simulink model "fft_block_3_19"  (R2023a)
settings: Solver=VariableStepAuto  StartTime=0.0  StopTime=1024*20  RelTol=1e-3
libraries: hdlsllib x7, dsphdlxfrm2 x2, HDLMathLib x2, simulink x1
settings Model: Creator=75549  LastModifiedBy=19595
settings ModelReferenceCC: EnableRefExpFcnMdlSchedulingChecks=on

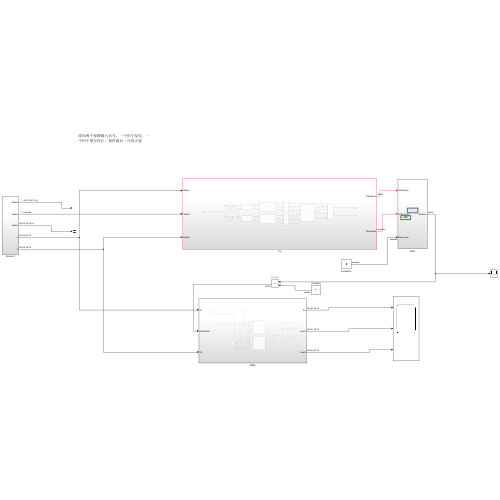
[thumbnail: Simulink's stored preview of the top-level diagram]
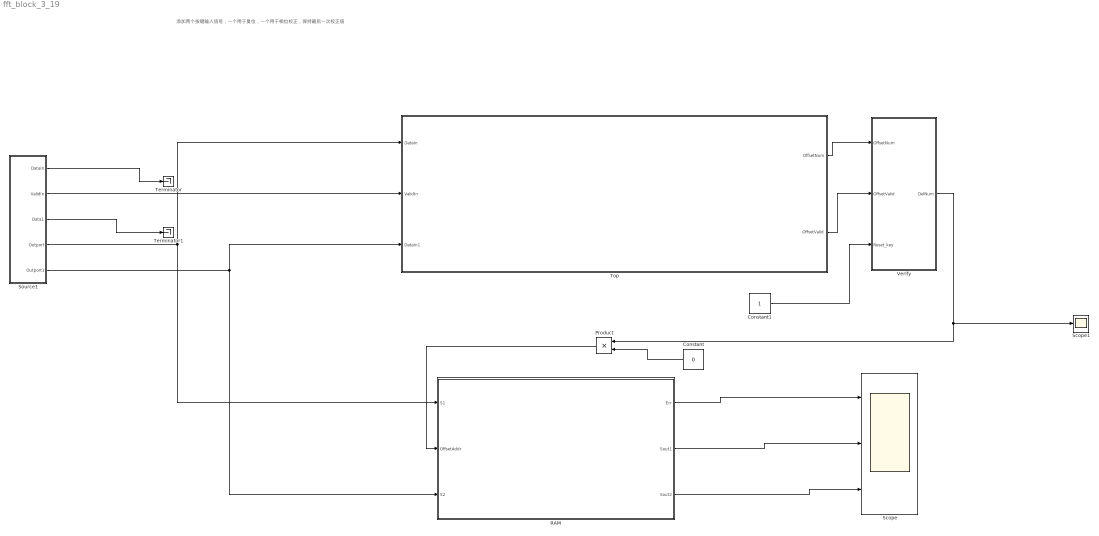
== system fft_block_3_19 ==
  note: 添加两个按键输入信号，一个用于复位，一个用于相位校正，保持最后一次校正值
  Constant : Constant  Value=0  VectorParams1D=off  SampleTime=-1
  Constant1 : Constant  VectorParams1D=off  OutDataTypeStr=boolean  SampleTime=-1
  Product : Product  OutDataTypeStr=uint16
  RAM : Subsystem
  Scope : Scope  NumInputPorts=3
  Scope1 : Scope
  Source1 : Subsystem
  Terminator : Terminator
  Terminator1 : Terminator
  Top : Subsystem
  Verify : Subsystem
  wires:
  Verify/1(DelNum) -> Product/1, Scope1/1
  RAM/2(Sout1) -> Scope/2
  Source1/4(Outport) -> Top/1(DataIn), RAM/1(S1)
  Source1/2(ValidIn) -> Top/2(ValidIn)
  Top/2(OffsetValid) -> Verify/2(OffsetValid)
  Top/1(OffsetNum) -> Verify/1(OffsetNum)
  Source1/1(DataIn) -> Terminator/1
  Source1/3(Data1) -> Terminator1/1
  RAM/1(Err) -> Scope/1
  Source1/5(Outport1) -> Top/3(DataIn1), RAM/3(S2)
  RAM/3(Sout2) -> Scope/3
  Constant/1 -> Product/2
  Product/1 -> RAM/2(OffsetAddr)
  Constant1/1 -> Verify/3(Reset_key)

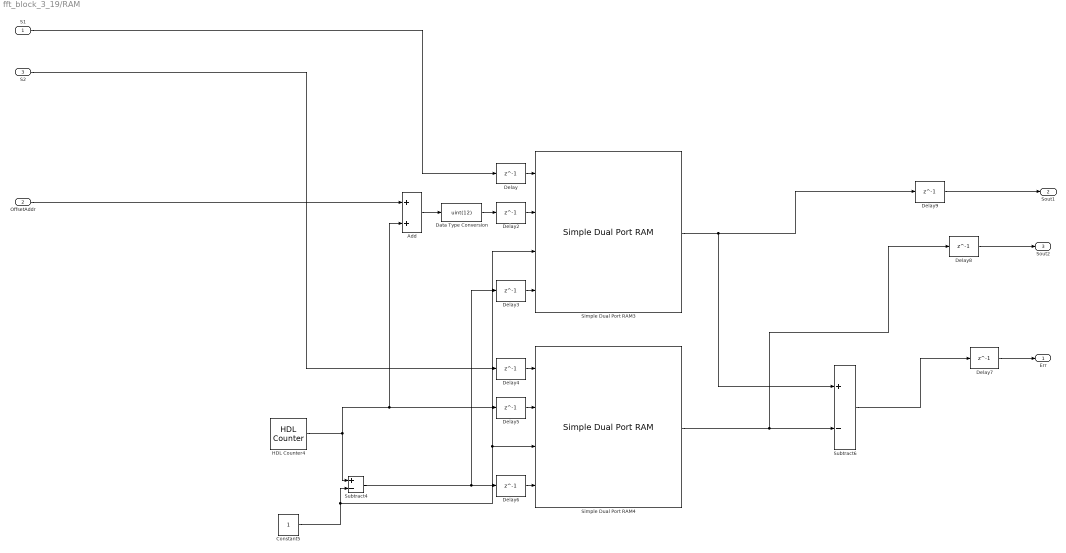
== system fft_block_3_19/RAM ==
  S1 : Inport
  OffsetAddr : Inport  Port=2
  S2 : Inport  Port=3
  Add : Sum  OutDataTypeStr=uint16
  Constant5 : Constant  VectorParams1D=off  OutDataTypeStr=Inherit: Inherit via back propagation  SampleTime=-1
  Data Type Conversion : DataTypeConversion  OutDataTypeStr=uint(12)  ConvertRealWorld=Stored Integer (SI)  SaturateOnIntegerOverflow=off  RndMeth=Floor
  Delay{,2..9} (9 alike) : Delay  DelayLength=1  InitialCondition=0  UseCircularBuffer=on
  HDL Counter4 : hdlsllib/Sources/HDL Counter  CountType=Count limited  CountInit=1  CountStep=1  CountMax=1024*4-1  CountFromType=Initial value  CountFrom=1  CountResetPort=off  CountLoadPort=off  CountEnbPort=off  CountDirPort=off  CountHitOutputPort=off  CountDataType=Unsigned  CountWordLen=12  CountFracLen=0  CountSampTime=1
  Simple Dual Port RAM3 : hdlsllib/HDL RAMs/Simple Dual Port RAM  ram_size=12
  Simple Dual Port RAM4 : hdlsllib/HDL RAMs/Simple Dual Port RAM  ram_size=12
  Subtract4 : Sum  Inputs=+-  OutDataTypeStr=uint(12)
  Subtract6 : Sum  Inputs=+-
  Err : Outport
  Sout1 : Outport  Port=2
  Sout2 : Outport  Port=3
  wires:
  S2/1 -> Delay4/1
  Constant5/1 -> Simple Dual Port RAM4/3, Simple Dual Port RAM3/3, Subtract4/2
  S1/1 -> Delay/1
  Simple Dual Port RAM3/1 -> Subtract6/1, Delay9/1
  Add/1 -> Data Type Conversion/1
  HDL Counter4/1 -> Add/2, Delay5/1, Subtract4/1
  Data Type Conversion/1 -> Delay2/1
  Simple Dual Port RAM4/1 -> Delay8/1, Subtract6/2
  Subtract6/1 -> Delay7/1
  OffsetAddr/1 -> Add/1
  Subtract4/1 -> Delay6/1, Delay3/1
  Delay/1 -> Simple Dual Port RAM3/1
  Delay2/1 -> Simple Dual Port RAM3/2
  Delay3/1 -> Simple Dual Port RAM3/4
  Delay4/1 -> Simple Dual Port RAM4/1
  Delay5/1 -> Simple Dual Port RAM4/2
  Delay6/1 -> Simple Dual Port RAM4/4
  Delay7/1 -> Err/1
  Delay8/1 -> Sout2/1
  Delay9/1 -> Sout1/1

== system fft_block_3_19/Source1 ==
  Subsystem : Subsystem
  DataIn : Outport  VectorParamsAs1DForOutWhenUnconnected=off
  ValidIn : Outport  Port=2  VectorParamsAs1DForOutWhenUnconnected=off
  Data1 : Outport  Port=3  VectorParamsAs1DForOutWhenUnconnected=off
  Outport : Outport  Port=4
  Outport1 : Outport  Port=5
  wires:
  Subsystem/3(vld) -> ValidIn/1
  Subsystem/1(Data) -> DataIn/1
  Subsystem/2(Data1) -> Data1/1
  Subsystem/4(Re1) -> Outport/1
  Subsystem/5(Re2) -> Outport1/1

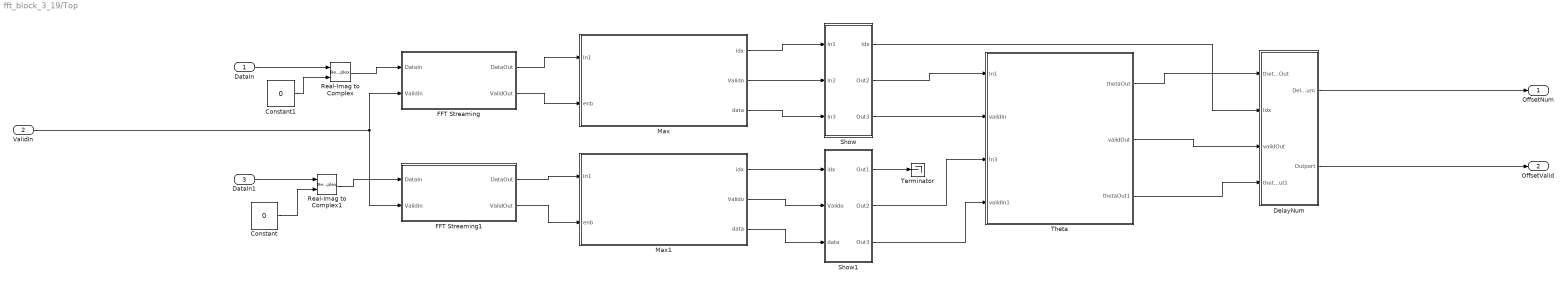
== system fft_block_3_19/Top ==
  DataIn : Inport
  ValidIn : Inport  Port=2
  DataIn1 : Inport  Port=3
  Constant : Constant  Value=0  VectorParams1D=off  OutDataTypeStr=Inherit: Inherit via back propagation  SampleTime=-1
  Constant1 : Constant  Value=0  VectorParams1D=off  OutDataTypeStr=Inherit: Inherit via back propagation  SampleTime=-1
  DelayNum : Subsystem
  FFT Streaming : Subsystem
  FFT Streaming1 : Subsystem
  Max : Subsystem
  Max1 : Subsystem
  Real-Imag to Complex : RealImagToComplex
  Real-Imag to Complex1 : RealImagToComplex
  Show : Subsystem
  Show1 : Subsystem
  Terminator : Terminator
  Theta : Subsystem
  OffsetNum : Outport
  OffsetValid : Outport  Port=2
  wires:
  ValidIn/1 -> FFT Streaming/2(ValidIn), FFT Streaming1/2(ValidIn)
  Max1/2(Valido) -> Show1/2(Valido)
  FFT Streaming1/2(ValidOut) -> Max1/2(enb)
  Max/2(Valido) -> Show/2(In2)
  FFT Streaming1/1(DataOut) -> Max1/1(In1)
  Max/3(data) -> Show/3(In3)
  Show/2(Out2) -> Theta/1(In1)
  Max/1(idx) -> Show/1(In1)
  Max1/1(idx) -> Show1/1(idx)
  Show1/3(Out3) -> Theta/4(validIn1)
  Max1/3(data) -> Show1/3(data)
  FFT Streaming/1(DataOut) -> Max/1(In1)
  FFT Streaming/2(ValidOut) -> Max/2(enb)
  DelayNum/1(DelayNum) -> OffsetNum/1
  Show1/2(Out2) -> Theta/3(In3)
  Show/3(Out3) -> Theta/2(validIn)
  Show1/1(Out1) -> Terminator/1
  Theta/1(thetaOut) -> DelayNum/1(thetaOut)
  Show/1(Idx) -> DelayNum/2(Idx)
  Theta/3(thetaOut1) -> DelayNum/4(thetaOut1)
  Theta/2(validOut) -> DelayNum/3(validOut)
  DelayNum/2(Outport) -> OffsetValid/1
  DataIn/1 -> Real-Imag to Complex/1
  DataIn1/1 -> Real-Imag to Complex1/1
  Real-Imag to Complex1/1 -> FFT Streaming1/1(DataIn)
  Constant/1 -> Real-Imag to Complex1/2
  Constant1/1 -> Real-Imag to Complex/2
  Real-Imag to Complex/1 -> FFT Streaming/1(DataIn)

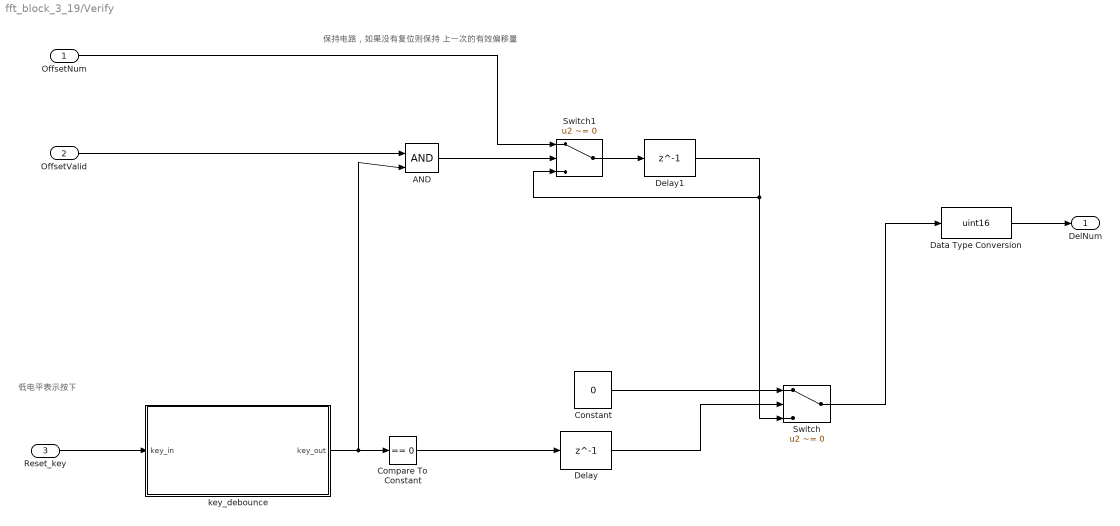
== system fft_block_3_19/Verify ==
  note: 保持电路，如果没有复位则保持 上一次的有效偏移量
  note: 低电平表示按下
  OffsetNum : Inport
  OffsetValid : Inport  Port=2
  Reset_key : Inport  Port=3  OutDataTypeStr=boolean
  AND : Logic  IconShape=distinctive  AllPortsSameDT=off  OutDataTypeStr=boolean
  Compare To Constant : hdlsllib/Logic and Bit Operations/Compare To Constant  relop===  const=0  OutDataTypeStr=boolean
  Constant : Constant  Value=0  VectorParams1D=off  OutDataTypeStr=int16  SampleTime=-1
  Data Type Conversion : DataTypeConversion  OutDataTypeStr=uint16  SaturateOnIntegerOverflow=off  RndMeth=Floor
  Delay : Delay  DelayLength=1  InitialCondition=0  UseCircularBuffer=on
  Delay1 : Delay  DelayLength=1  InitialCondition=0  UseCircularBuffer=on
  Switch : Switch  Criteria=u2 ~= 0  SaturateOnIntegerOverflow=off  InputSameDT=off
  Switch1 : Switch  Criteria=u2 ~= 0  SaturateOnIntegerOverflow=off  InputSameDT=off
  key_debounce : Subsystem
  DelNum : Outport
  wires:
  Reset_key/1 -> key_debounce/1(key_in)
  key_debounce/1(key_out) -> AND/2, Compare To Constant/1
  Data Type Conversion/1 -> DelNum/1
  Compare To Constant/1 -> Delay/1
  Constant/1 -> Switch/1
  OffsetValid/1 -> AND/1
  AND/1 -> Switch1/2
  OffsetNum/1 -> Switch1/1
  Switch1/1 -> Delay1/1
  Delay1/1 -> Switch/3, Switch1/3
  Switch/1 -> Data Type Conversion/1
  Delay/1 -> Switch/2

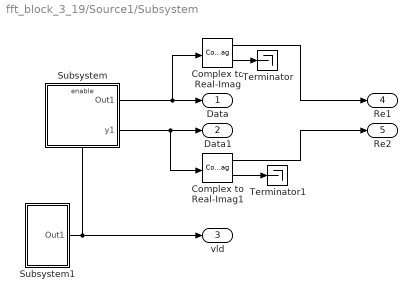
== system fft_block_3_19/Source1/Subsystem ==
  Complex to Real-Imag : ComplexToRealImag
  Complex to Real-Imag1 : ComplexToRealImag
  Subsystem : Subsystem
  Subsystem1 : Subsystem
  Terminator : Terminator
  Terminator1 : Terminator
  Data : Outport  VectorParamsAs1DForOutWhenUnconnected=off
  Data1 : Outport  Port=2  VectorParamsAs1DForOutWhenUnconnected=off
  vld : Outport  Port=3  VectorParamsAs1DForOutWhenUnconnected=off
  Re1 : Outport  Port=4  VectorParamsAs1DForOutWhenUnconnected=off
  Re2 : Outport  Port=5  VectorParamsAs1DForOutWhenUnconnected=off
  wires:
  Subsystem1/1(Out1) -> vld/1, Subsystem/Enable
  Subsystem/1(Out1) -> Complex to Real-Imag/1, Data/1
  Subsystem/2(y1) -> Complex to Real-Imag1/1, Data1/1
  Complex to Real-Imag/1 -> Re1/1
  Complex to Real-Imag1/1 -> Re2/1
  Complex to Real-Imag/2 -> Terminator/1
  Complex to Real-Imag1/2 -> Terminator1/1

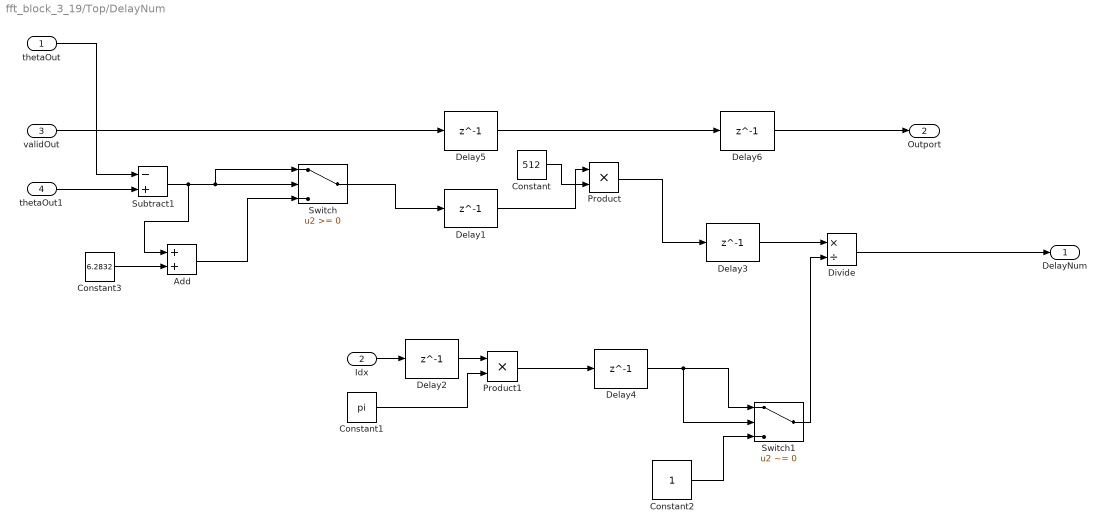
== system fft_block_3_19/Top/DelayNum ==
  thetaOut : Inport
  Idx : Inport  Port=2
  validOut : Inport  Port=3
  thetaOut1 : Inport  Port=4
  Add : Sum
  Constant : Constant  Value=512  OutDataTypeStr=uint16  SampleTime=-1
  Constant1 : Constant  Value=pi  VectorParams1D=off  OutDataTypeStr=fixdt(1,17,13)  SampleTime=-1
  Constant2 : Constant  VectorParams1D=off  OutDataTypeStr=fixdt(1,27,13)  SampleTime=-1
  Constant3 : Constant  Value=6.2832  VectorParams1D=off  OutDataTypeStr=fixdt(1,17,13)  SampleTime=-1
  Delay{1..6} (6 alike) : Delay  DelayLength=1  InitialCondition=0  UseCircularBuffer=on
  Divide : Product  Inputs=*/  RndMeth=Simplest  SaturateOnIntegerOverflow=on
  Product : Product
  Product1 : Product
  Subtract1 : Sum  Inputs=-+
  Switch : Switch  SaturateOnIntegerOverflow=off  InputSameDT=off
  Switch1 : Switch  Criteria=u2 ~= 0  SaturateOnIntegerOverflow=off  InputSameDT=off
  DelayNum : Outport  InitialOutput=0
  Outport : Outport  Port=2
  wires:
  Constant/1 -> Product/2
  Idx/1 -> Delay2/1
  Constant1/1 -> Product1/2
  Product/1 -> Delay3/1
  thetaOut1/1 -> Subtract1/2
  thetaOut/1 -> Subtract1/1
  Subtract1/1 -> Add/1, Switch/1, Switch/2
  Product1/1 -> Delay4/1
  Divide/1 -> DelayNum/1
  Delay1/1 -> Product/1
  Delay2/1 -> Product1/1
  Delay3/1 -> Divide/1
  Delay4/1 -> Switch1/2, Switch1/1
  validOut/1 -> Delay5/1
  Delay5/1 -> Delay6/1
  Delay6/1 -> Outport/1
  Constant2/1 -> Switch1/3
  Switch1/1 -> Divide/2
  Add/1 -> Switch/3
  Switch/1 -> Delay1/1
  Constant3/1 -> Add/2

== system fft_block_3_19/Top/FFT Streaming ==
  note: FFT单元，输入输出添加了寄存器
  DataIn : Inport
  ValidIn : Inport  Port=2
  Delay{,1..3} (4 alike) : Delay  DelayLength=1  InitialCondition=0  UseCircularBuffer=on
  FFT : dsphdlxfrm2/FFT  FFTLength=1024  Architecture=Streaming Radix 2^2  ComplexMultiplication=Use 4 multipliers and 2 adders  BitReversedOutput=off  BitReversedInput=off  Normalize=on  SimulateUsing=Code generation  RoundingMethod=Floor  ResetInputPort=off  StartOutputPort=off  EndOutputPort=off
  DataOut : Outport  VectorParamsAs1DForOutWhenUnconnected=off
  ValidOut : Outport  Port=2  VectorParamsAs1DForOutWhenUnconnected=off
  wires:
  DataIn/1 -> Delay/1
  ValidIn/1 -> Delay1/1
  FFT/1 -> Delay2/1
  FFT/2 -> Delay3/1
  Delay/1 -> FFT/1
  Delay1/1 -> FFT/2
  Delay2/1 -> DataOut/1
  Delay3/1 -> ValidOut/1

== system fft_block_3_19/Top/FFT Streaming1 ==
  DataIn : Inport
  ValidIn : Inport  Port=2
  Delay{,1..3} (4 alike) : Delay  DelayLength=1  InitialCondition=0  UseCircularBuffer=on
  FFT : dsphdlxfrm2/FFT  FFTLength=1024  Architecture=Streaming Radix 2^2  ComplexMultiplication=Use 4 multipliers and 2 adders  BitReversedOutput=off  BitReversedInput=off  Normalize=on  SimulateUsing=Code generation  RoundingMethod=Floor  ResetInputPort=off  StartOutputPort=off  EndOutputPort=off
  DataOut : Outport  VectorParamsAs1DForOutWhenUnconnected=off
  ValidOut : Outport  Port=2  VectorParamsAs1DForOutWhenUnconnected=off
  wires:
  DataIn/1 -> Delay/1
  ValidIn/1 -> Delay1/1
  FFT/1 -> Delay2/1
  FFT/2 -> Delay3/1
  Delay/1 -> FFT/1
  Delay1/1 -> FFT/2
  Delay2/1 -> DataOut/1
  Delay3/1 -> ValidOut/1

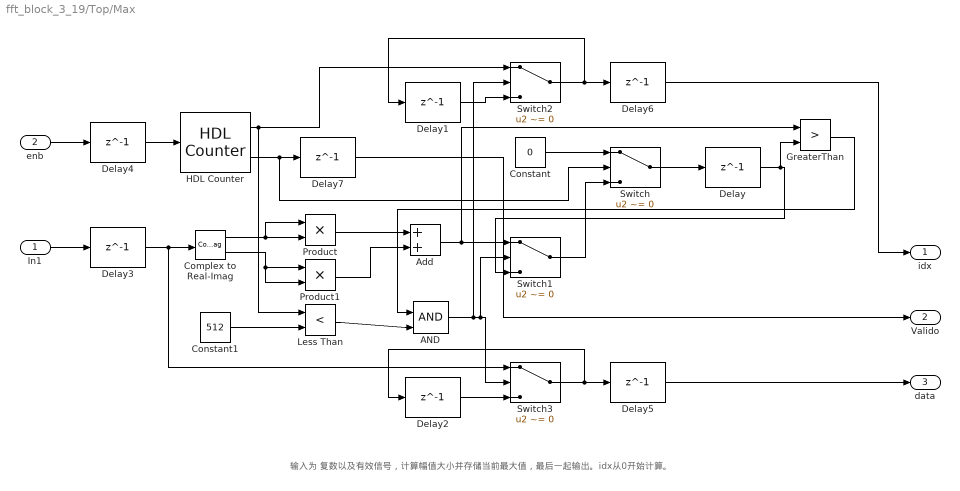
== system fft_block_3_19/Top/Max ==
  note: 输入为 复数以及有效信号，计算幅值大小并存储当前最大值，最后一起输出。idx从0开始计算。
  In1 : Inport
  enb : Inport  Port=2
  AND : Logic  IconShape=distinctive  AllPortsSameDT=off  OutDataTypeStr=boolean
  Add : Sum
  Complex to Real-Imag : ComplexToRealImag
  Constant : Constant  Value=0  VectorParams1D=off  OutDataTypeStr=Inherit: Inherit via back propagation  SampleTime=-1
  Constant1 : Constant  Value=512  VectorParams1D=off  OutDataTypeStr=Inherit: Inherit via back propagation  SampleTime=-1
  Delay{,1..7} (8 alike) : Delay  DelayLength=1  InitialCondition=0  UseCircularBuffer=on
  GreaterThan : RelationalOperator  Operator=>  OutDataTypeStr=boolean  RndMeth=Simplest  InputSameDT=off
  HDL Counter : hdlsllib/Sources/HDL Counter  CountType=Count limited  CountInit=0  CountStep=1  CountMax=1023  CountFromType=Initial value  CountFrom=0  CountResetPort=off  CountLoadPort=off  CountEnbPort=on  CountDirPort=off  CountHitOutputPort=on  CountDataType=Unsigned  CountWordLen=10  CountFracLen=0  CountSampTime=1
  Less Than : RelationalOperator  Operator=<  OutDataTypeStr=boolean  RndMeth=Simplest  InputSameDT=off
  Product : Product
  Product1 : Product
  Switch{,1..3} (4 alike) : Switch  Criteria=u2 ~= 0  SaturateOnIntegerOverflow=off  InputSameDT=off
  idx : Outport
  Valido : Outport  Port=2
  data : Outport  Port=3
  wires:
  Delay7/1 -> Valido/1
  Switch2/1 -> Delay1/1, Delay6/1
  Delay5/1 -> data/1
  Delay6/1 -> idx/1
  HDL Counter/1 -> Switch2/1, Less Than/1
  Delay4/1 -> HDL Counter/1
  Delay2/1 -> Switch3/3
  GreaterThan/1 -> AND/1
  Less Than/1 -> AND/2
  Constant1/1 -> Less Than/2
  Delay1/1 -> Switch2/3
  enb/1 -> Delay4/1
  Product/1 -> Add/1
  Switch1/1 -> Switch/3
  Switch/1 -> Delay/1
  Complex to Real-Imag/2 -> Product1/2, Product1/1
  Constant/1 -> Switch/1
  In1/1 -> Delay3/1
  Product1/1 -> Add/2
  Delay3/1 -> Complex to Real-Imag/1, Switch3/1
  Switch3/1 -> Delay2/1, Delay5/1
  AND/1 -> Switch1/2, Switch3/2, Switch2/2
  HDL Counter/2 -> Switch/2, Delay7/1
  Delay/1 -> GreaterThan/2, Switch1/3
  Add/1 -> GreaterThan/1, Switch1/1
  Complex to Real-Imag/1 -> Product/2, Product/1

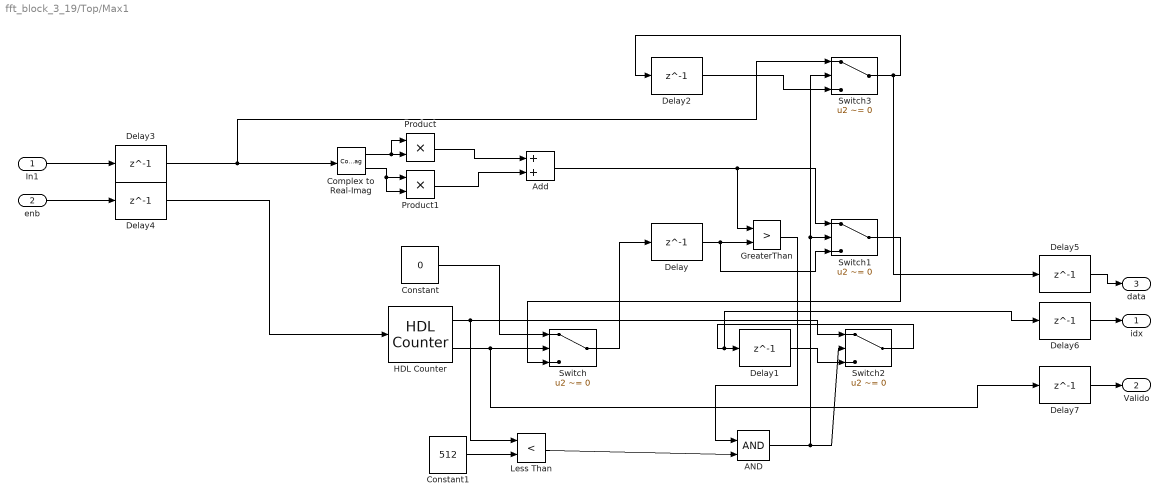
== system fft_block_3_19/Top/Max1 ==
  In1 : Inport
  enb : Inport  Port=2
  AND : Logic  IconShape=distinctive  AllPortsSameDT=off  OutDataTypeStr=boolean
  Add : Sum
  Complex to Real-Imag : ComplexToRealImag
  Constant : Constant  Value=0  VectorParams1D=off  OutDataTypeStr=Inherit: Inherit via back propagation  SampleTime=-1
  Constant1 : Constant  Value=512  VectorParams1D=off  OutDataTypeStr=Inherit: Inherit via back propagation  SampleTime=-1
  Delay{,1..7} (8 alike) : Delay  DelayLength=1  InitialCondition=0  UseCircularBuffer=on
  GreaterThan : RelationalOperator  Operator=>  OutDataTypeStr=boolean  RndMeth=Simplest  InputSameDT=off
  HDL Counter : hdlsllib/Sources/HDL Counter  CountType=Count limited  CountInit=0  CountStep=1  CountMax=1023  CountFromType=Initial value  CountFrom=0  CountResetPort=off  CountLoadPort=off  CountEnbPort=on  CountDirPort=off  CountHitOutputPort=on  CountDataType=Unsigned  CountWordLen=10  CountFracLen=0  CountSampTime=1
  Less Than : RelationalOperator  Operator=<  OutDataTypeStr=boolean  RndMeth=Simplest  InputSameDT=off
  Product : Product
  Product1 : Product
  Switch{,1..3} (4 alike) : Switch  Criteria=u2 ~= 0  SaturateOnIntegerOverflow=off  InputSameDT=off
  idx : Outport
  Valido : Outport  Port=2
  data : Outport  Port=3
  wires:
  Complex to Real-Imag/1 -> Product/1, Product/2
  Product1/1 -> Add/2
  Add/1 -> Switch1/1, GreaterThan/1
  Delay/1 -> Switch1/3, GreaterThan/2
  In1/1 -> Delay3/1
  Constant/1 -> Switch/1
  Complex to Real-Imag/2 -> Product1/1, Product1/2
  Switch/1 -> Delay/1
  Switch1/1 -> Switch/3
  HDL Counter/2 -> Delay7/1, Switch/2
  Product/1 -> Add/1
  enb/1 -> Delay4/1
  Delay1/1 -> Switch2/3
  HDL Counter/1 -> Less Than/1, Switch2/1
  Switch2/1 -> Delay6/1, Delay1/1
  Constant1/1 -> Less Than/2
  Less Than/1 -> AND/2
  GreaterThan/1 -> AND/1
  AND/1 -> Switch3/2, Switch1/2, Switch2/2
  Delay2/1 -> Switch3/3
  Switch3/1 -> Delay5/1, Delay2/1
  Delay3/1 -> Complex to Real-Imag/1, Switch3/1
  Delay4/1 -> HDL Counter/1
  Delay5/1 -> data/1
  Delay6/1 -> idx/1
  Delay7/1 -> Valido/1

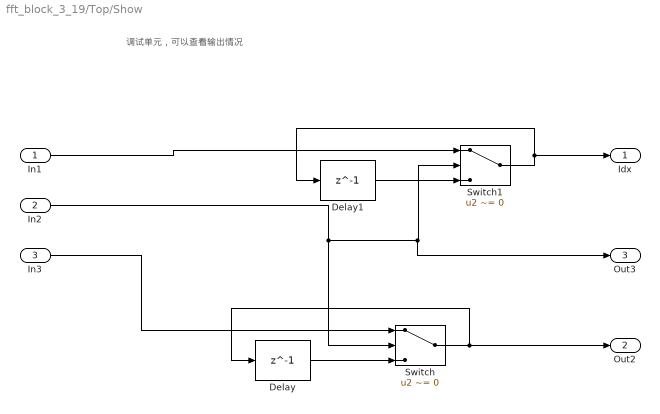
== system fft_block_3_19/Top/Show ==
  note: 调试单元，可以查看输出情况
  In1 : Inport
  In2 : Inport  Port=2
  In3 : Inport  Port=3
  Delay : Delay  DelayLength=1  InitialCondition=0  UseCircularBuffer=on
  Delay1 : Delay  DelayLength=1  InitialCondition=0  UseCircularBuffer=on
  Switch : Switch  Criteria=u2 ~= 0  SaturateOnIntegerOverflow=off  InputSameDT=off
  Switch1 : Switch  Criteria=u2 ~= 0  SaturateOnIntegerOverflow=off  InputSameDT=off
  Idx : Outport
  Out2 : Outport  Port=2
  Out3 : Outport  Port=3
  wires:
  Switch/1 -> Delay/1, Out2/1
  Delay/1 -> Switch/3
  Switch1/1 -> Idx/1, Delay1/1
  In3/1 -> Switch/1
  Delay1/1 -> Switch1/3
  In2/1 -> Out3/1, Switch1/2, Switch/2
  In1/1 -> Switch1/1

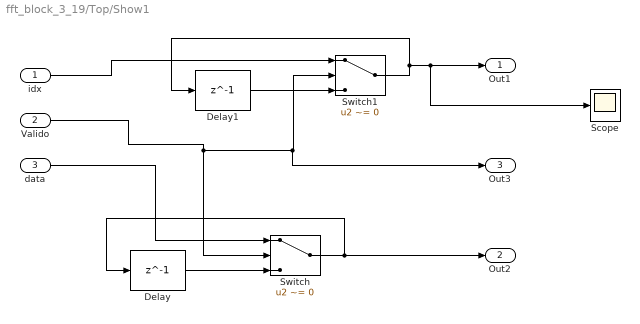
== system fft_block_3_19/Top/Show1 ==
  idx : Inport
  Valido : Inport  Port=2
  data : Inport  Port=3
  Delay : Delay  DelayLength=1  InitialCondition=0  UseCircularBuffer=on
  Delay1 : Delay  DelayLength=1  InitialCondition=0  UseCircularBuffer=on
  Scope : Scope
  Switch : Switch  Criteria=u2 ~= 0  SaturateOnIntegerOverflow=off  InputSameDT=off
  Switch1 : Switch  Criteria=u2 ~= 0  SaturateOnIntegerOverflow=off  InputSameDT=off
  Out1 : Outport
  Out2 : Outport  Port=2
  Out3 : Outport  Port=3
  wires:
  Switch/1 -> Delay/1, Out2/1
  Delay/1 -> Switch/3
  Switch1/1 -> Scope/1, Out1/1, Delay1/1
  data/1 -> Switch/1
  Delay1/1 -> Switch1/3
  Valido/1 -> Out3/1, Switch1/2, Switch/2
  idx/1 -> Switch1/1

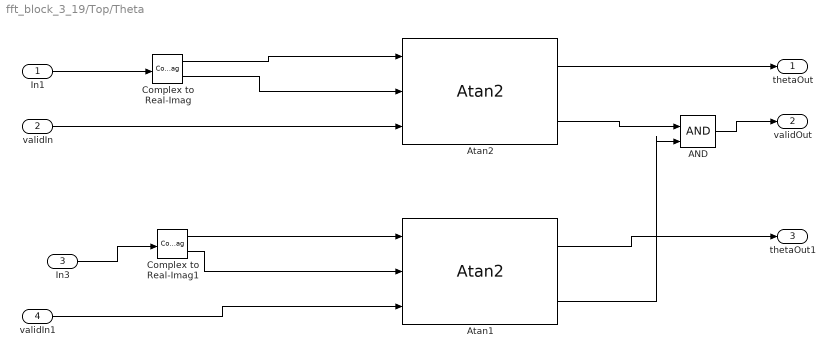
== system fft_block_3_19/Top/Theta ==
  In1 : Inport
  validIn : Inport  Port=2
  In3 : Inport  Port=3
  validIn1 : Inport  Port=4
  AND : Logic  IconShape=distinctive  AllPortsSameDT=off  OutDataTypeStr=boolean
  Atan1 : HDLMathLib/Atan2  iter=11  latencyMode=Max  customLatencyValue=0
  Atan2 : HDLMathLib/Atan2  iter=11  latencyMode=Max  customLatencyValue=0
  Complex to Real-Imag : ComplexToRealImag
  Complex to Real-Imag1 : ComplexToRealImag
  thetaOut : Outport
  validOut : Outport  Port=2
  thetaOut1 : Outport  Port=3
  wires:
  Atan1/1 -> thetaOut1/1
  Complex to Real-Imag/2 -> Atan2/2
  Complex to Real-Imag1/1 -> Atan1/1
  Complex to Real-Imag1/2 -> Atan1/2
  Complex to Real-Imag/1 -> Atan2/1
  In1/1 -> Complex to Real-Imag/1
  validIn/1 -> Atan2/3
  validIn1/1 -> Atan1/3
  In3/1 -> Complex to Real-Imag1/1
  Atan1/2 -> AND/2
  Atan2/1 -> thetaOut/1
  Atan2/2 -> AND/1
  AND/1 -> validOut/1

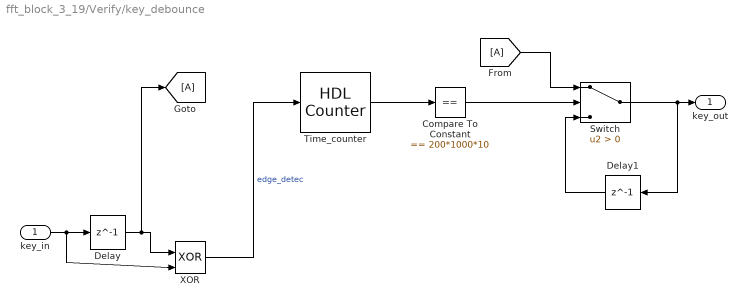
== system fft_block_3_19/Verify/key_debounce ==
  key_in : Inport
  Compare To Constant : simulink/Logic and Bit Operations/Compare To Constant  relop===  const=200*1000*10  OutDataTypeStr=boolean
  Delay : Delay  DelayLength=1  InitialCondition=1
  Delay1 : Delay  DelayLength=1  InitialCondition=1
  From : From
  Goto : Goto
  Switch : Switch  Criteria=u2 > Threshold  SaturateOnIntegerOverflow=off  InputSameDT=off
  Time_counter : hdlsllib/Sources/HDL Counter  CountType=Count limited  CountInit=0  CountStep=1  CountMax=200*1000*10  CountFromType=Initial value  CountFrom=0  CountResetPort=on  CountLoadPort=off  CountEnbPort=off  CountDirPort=off  CountHitOutputPort=off  CountDataType=Unsigned  CountWordLen=32  CountFracLen=0  CountSampTime=1
  XOR : Logic  Operator=XOR  IconShape=distinctive  AllPortsSameDT=off  OutDataTypeStr=boolean
  key_out : Outport  VectorParamsAs1DForOutWhenUnconnected=off
  wires:
  key_in/1 -> XOR/2, Delay/1
  Delay/1 -> Goto/1, XOR/1
  XOR/1 -> Time_counter/1  "edge_detec"
  Time_counter/1 -> Compare To Constant/1
  Switch/1 -> Delay1/1, key_out/1
  Compare To Constant/1 -> Switch/2
  From/1 -> Switch/1
  Delay1/1 -> Switch/3

== system fft_block_3_19/Source1/Subsystem/Subsystem ==
  Enable : EnablePort
  Data Source : MATLAB Function  TreatAsAtomicUnit=on
  Out1 : Outport  VectorParamsAs1DForOutWhenUnconnected=off
  y1 : Outport  Port=2  VectorParamsAs1DForOutWhenUnconnected=off
  wires:
  Data Source/1(y) -> Out1/1
  Data Source/2(y1) -> y1/1

== system fft_block_3_19/Source1/Subsystem/Subsystem1 ==
  Constant : Constant  Value=[1 0 ]  OutDataTypeStr=boolean  SampleTime=-1
  Unbuffer : Unbuffer
  Out1 : Outport  VectorParamsAs1DForOutWhenUnconnected=off
  wires:
  Constant/1 -> Unbuffer/1
  Unbuffer/1 -> Out1/1

== matlab function fft_block_3_19/Source1/Subsystem/Subsystem/Data Source ==
  settings: updateMethod=DISCRETE  sampleTime=1
  data: y output; y1 output
function [y,y1] = fcn()
Fs  = 650e6;
FrameSize  = 1;
persistent sinegen1 
persistent sinegen2
noiseVar   = 0;
% 信号频率实际为 2.5e6
if isempty(sinegen1)
    sinegen1 = dsp.SineWave('Amplitude', 1, 'Frequency',6.5e6, 'SampleRate',Fs,'SamplesPerFrame',FrameSize,'PhaseOffset',pi/5);
    sinegen2 = dsp.SineWave('Amplitude', 1, 'Frequency',6.5e6, 'SampleRate',Fs,'SamplesPerFrame',FrameSize);

end

y = complex(fi(sinegen1() + sqrt(noiseVar)*randn(FrameSize,1), 1, 16, 13));
y1 = complex(fi(sinegen2() + sqrt(noiseVar)*randn(FrameSize,1), 1, 16, 13));
